simulink model "section_4_1_1"  (R2021b)
settings: Solver=VariableStepAuto  StartTime=0.0  StopTime=2000  RelTol=1e-3
values from neighbouring files (symbols this model uses):
  Cz_den = cell2mat(Cz.Denominator)    [lab3.m]
  Cz_num = cell2mat(Cz.Numerator)    [lab3.m]
  K = 1e-5    (= 1e-05)    [lab3.m]
  Pz_den = cell2mat(Pz.Denominator)    [lab3.m]
  Pz_num = cell2mat(Pz.Numerator)    [lab3.m]
  T = 0.1    [lab3.m]
settings Model: Creator=varunsampat  LastModifiedBy=varunsampat

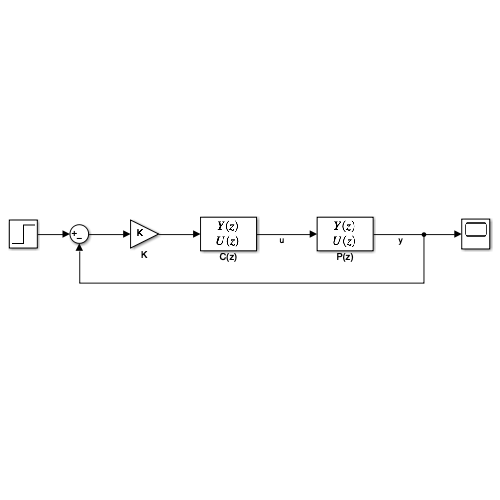
[thumbnail: Simulink's stored preview of the top-level diagram]
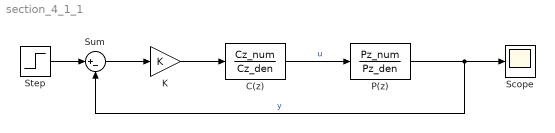
== system section_4_1_1 ==
  C(z) : DiscreteTransferFcn  Numerator=Cz_num  Denominator=Cz_den
  K : Gain  Gain=K
  P(z) : DiscreteTransferFcn  Numerator=Pz_num  Denominator=Pz_den
  Scope : Scope
  Step : Step  SampleTime=T
  Sum : Sum  Inputs=|+-
  wires:
  C(z)/1 -> P(z)/1  "u"
  K/1 -> C(z)/1
  Sum/1 -> K/1
  P(z)/1 -> Sum/2, Scope/1  "y"
  Step/1 -> Sum/1
